simulink model "FlightAngCntrlSimulink"  (R2015a)
settings: Solver=ode8  StartTime=0.0  StopTime=10.0  RelTol=1e-3
values from neighbouring files (symbols this model uses):
  ConversionFactor = 1000    [FlightAngCntrlBlackBox.m]
  IGain = 0    [FlightAngCntrlBlackBox.m]
  MinThrust = 8000    [FlightAngCntrlBlackBox.m]
  PGain = 1    [FlightAngCntrlBlackBox.m]
  RefThetha = 0    [FlightAngCntrlBlackBox.m]
  SlopeOfCurve = 2000    [FlightAngCntrlBlackBox.m]
  TimeConstant = 1    [FlightAngCntrlBlackBox.m]
undefined symbols (not defined in the file or in its folder): sigbuilder_block
libraries: simulink x1
settings Model: Creator=kshenoy  LastModifiedBy=kshenoy

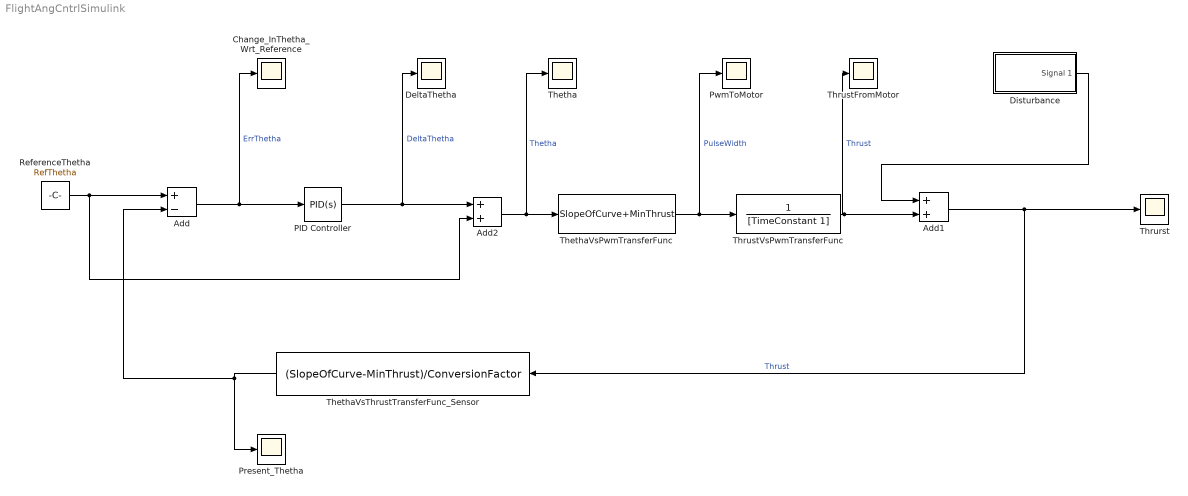
== system FlightAngCntrlSimulink ==
  Add : Sum  Inputs=+-
  Add1 : Sum
  Add2 : Sum
  Change_InThetha_Wrt_Reference : Scope
      settings: SaveName=ScopeData4
  DeltaThetha : Scope
      settings: SaveName=ScopeData5
  Disturbance : Subsystem  Tag=STV Subsys  LoadFcn=sigbuilder_block('load');  StartFcn=sigbuilder_block('start');  StopFcn=sigbuilder_block('stop');  ClipboardFcn=sigbuilder_block('clipboard');  mask(Sigbuilder block){}
      mask help: Simulink:masks:SigbuilderBlock_MD
      mask init:
      | if ~strcmp(get_param(bdroot(gcbh),'SimulationStatus'),'stopped') tuvar = sigbuilder_block('maskInit'); end
      settings: CopyFcn=sigbuilder_block('copy');  DeleteFcn=sigbuilder_block('delete');  ModelCloseFcn=sigbuilder_block('modelClose');  PreSaveFcn=sigbuilder_block('preSave');  PauseFcn=sigbuilder_block('pause');  ContinueFcn=sigbuilder_block('continue');  NameChangeFcn=sigbuilder_block('namechange');  OpenFcn=sigbuilder_block('open',[437.6 199.2 550.4 400 ]);  CloseFcn=sigbuilder_block('close');
      mask Display: plot(0, 0, 100, 100,[2, 2, 32, 32, 2], [68, 8, 8, 68, 68],[32, 2], [38, 38], [32, 19, 2],[53, 60, 44], [32, 17, 17, 2],[16, 16, 31, 31]);txt = getActiveGroup(gcbh);text(2, 100, txt,'verticalAlignment', 'top');
  PID Controller : simulink/Continuous/PID Controller  Controller=PID  TimeDomain=Continuous-time  SampleTime=-1  IntegratorMethod=Forward Euler  FilterMethod=Forward Euler  Form=Ideal  UseFilter=on  ControllerParametersSource=internal  P=PGain  I=IGain  D=0  N=100  InitialConditionSource=internal  InitialConditionForIntegrator=0  InitialConditionForFilter=0  ExternalReset=none  LimitOutput=off  UpperSaturationLimit=inf  LowerSaturationLimit=-inf  LinearizeAsGain=on  AntiWindupMode=none  Kb=1  TrackingMode=off  Kt=1  PParamMin=[]  PParamMax=[]  IParamMin=[]  IParamMax=[]  DParamMin=[]  DParamMax=[]  NParamMin=[]  NParamMax=[]  KbParamMin=[]  KbParamMax=[]  KtParamMin=[]  KtParamMax=[]  POutMin=[]  POutMax=[]  IOutMin=[]  IOutMax=[]  DOutMin=[]  DOutMax=[]  NOutMin=[]  NOutMax=[]  KbOutMin=[]  KbOutMax=[]  KtOutMin=[]  KtOutMax=[]  IntegratorOutMin=[]  IntegratorOutMax=[]  FilterOutMin=[]  FilterOutMax=[]  SumOutMin=[]  SumOutMax=[]  SumI1OutMin=[]  SumI1OutMax=[]  SumI2OutMin=[]  SumI2OutMax=[]  SumI3OutMin=[]  SumI3OutMax=[]  SumDOutMin=[]  SumDOutMax=[]  SaturationOutMin=[]  SaturationOutMax=[]  IntegratorContinuousStateAttributes=''  IntegratorStateMustResolveToSignalObject=off  IntegratorRTWStateStorageClass=Auto  FilterContinuousStateAttributes=''  FilterStateMustResolveToSignalObject=off  FilterRTWStateStorageClass=Auto  DifferentiatorICPrevScaledInput=0  DifferentiatorOutMin=[]  DifferentiatorOutMax=[]
  Present_Thetha : Scope
      settings: SaveName=ScopeData3
  PwmToMotor : Scope
  ReferenceThetha : Constant  Value=RefThetha
  Thetha : Scope
      settings: SaveName=ScopeData2
  ThethaVsPwmTransferFunc : Fcn  Expr=SlopeOfCurve+MinThrust
  ThethaVsThrustTransferFunc_Sensor : Fcn  Expr=(SlopeOfCurve-MinThrust)/ConversionFactor
  Thrurst : Scope
      settings: TimeRange=10  YMin=0  YMax=8000
  ThrustFromMotor : Scope
      settings: TimeRange=10  YMin=0  YMax=8000  SaveName=ScopeData6
  ThrustVsPwmTransferFunc : TransferFcn  Denominator=[TimeConstant 1]
  wires:
  Add/1 -> Change_InThetha_Wrt_Reference/1, PID Controller/1  "ErrThetha"
  ReferenceThetha/1 -> Add/1, Add2/2
  ThrustVsPwmTransferFunc/1 -> ThrustFromMotor/1, Add1/2  "Thrust"
  Disturbance/1(Signal 1) -> Add1/1
  Add1/1 -> ThethaVsThrustTransferFunc_Sensor/1, Thrurst/1  "Thrust"
  ThethaVsThrustTransferFunc_Sensor/1 -> Present_Thetha/1, Add/2
  PID Controller/1 -> DeltaThetha/1, Add2/1  "DeltaThetha"
  Add2/1 -> Thetha/1, ThethaVsPwmTransferFunc/1  "Thetha"
  ThethaVsPwmTransferFunc/1 -> PwmToMotor/1, ThrustVsPwmTransferFunc/1  "PulseWidth"

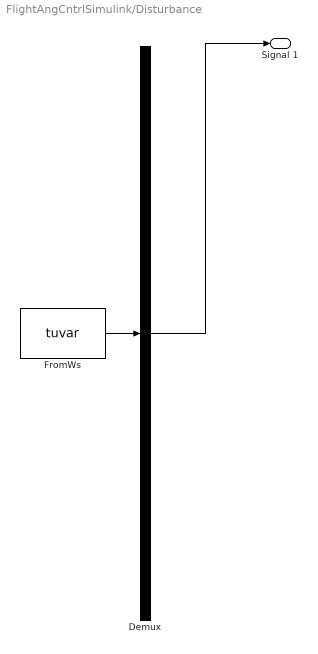
== system FlightAngCntrlSimulink/Disturbance ==
  Demux : Demux  Tag=STV Demux  Outputs=1
  FromWs : FromWorkspace  Tag=STV FromWs  VariableName=tuvar  SampleTime=0
      SigBuilderData=|
      | common.afterFinalStr = 'Extrapolate'
      | common.sampleTime = 0
      | dataSet.timeRange = [0 10]
      | dataSet.name = 'Group 1'
      | sbobj.Groups.Name = 'Group 1'
      | sbobj.Groups.Signals.Name = 'Signal 1'
      | sbobj.Groups.Signals.XData = [0 4 4 6 6 10]
      | sbobj.Groups.Signals.YData = [0 0 4920 4920 0 0]
  Signal 1 : Outport  Tag=STV Outport
  wires:
  Demux/1 -> Signal 1/1
  FromWs/1 -> Demux/1
